simulink model "HoppingLEGSimple"  (Simulink 7.7)
settings: Solver=ode3  StartTime=0.0  StopTime=5  FixedStep=0.001  RelTol=1e-3
settings Model: Creator=Alan Mutka  LastModifiedBy=Alan Mutka

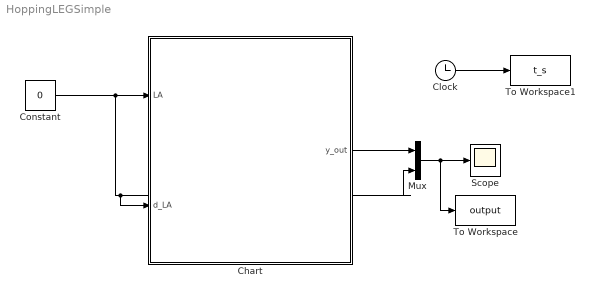
== system HoppingLEGSimple ==
  Chart : Stateflow chart  TreatAsAtomicUnit=on
  Clock : Clock
      settings: Decimation=10
  Constant : Constant  Value=0
  Mux : Mux  Inputs=2
  Scope : Scope
      settings: TimeRange=9.9  YMin=-0.5  YMax=8
  To Workspace : ToWorkspace  VariableName=output  SampleTime=0.001  SaveFormat=Array
  To Workspace1 : ToWorkspace  VariableName=t_s  SampleTime=0.001  SaveFormat=Array
  wires:
  Chart/1(y_out) -> Mux/1
  Mux/1 -> Scope/1, To Workspace/1
  Clock/1 -> To Workspace1/1
  Constant/1 -> Chart/1(LA), Mux/2, Chart/2(d_LA)

== stateflow chart Chart ==
  settings: updateMethod=CONTINUOUS
  state Stancedown
    du:
    l_dot = lv;
    lv_dot =k/mass*(l0+LA-l)-9.81-c/mass*lv+c/mass*d_LA;
    y_out = l;
  (default) -> Stancedown : {
      | l=0;lv= -7.0441;
      | }
  data: l local double; yv local double; y_out output double; y local double; lv local double; k constant double =30; mass constant double =1; l0 constant double =0; c constant double =1; LA input double =0; d_LA input double =0
  data l settings: updateMethod=SF_CONTINUOUS_TIME_DATA
  data yv settings: updateMethod=SF_CONTINUOUS_TIME_DATA
  data y settings: updateMethod=SF_CONTINUOUS_TIME_DATA
  data lv settings: updateMethod=SF_CONTINUOUS_TIME_DATA
